simulink model "IP_order1_math_model"  (R2021a)
settings: Solver=FixedStepAuto  StartTime=0.0  StopTime=10  FixedStep=1e-4  RelTol=1e-4
values from neighbouring files (symbols this model uses):
  g = 9.8    [main_order1.m]
  I = m*l^2/3    (= 0.0166666666667)    [main_order1.m]
  K = K_lqr    [main_order1.m]
  K_lqr = lqr(A,B,Q,R)    [main_order1.m]
  l = 0.5    [main_order1.m]
  m = A_k * m +C_k    [SolveLinearMPC.m]    (also in main_order1.m = 0.2)
  M = cell2mat(M)    [SolveLinearMPC.m]    (also in main_order1.m = 0.6)
libraries: pid_lib x2
settings Model: Creator=cc  LastModifiedBy=zyinx

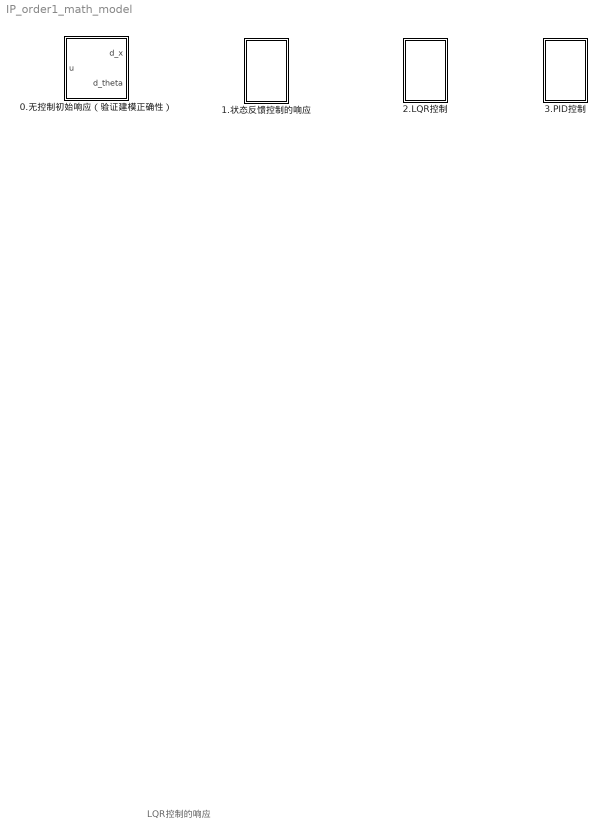
== system IP_order1_math_model ==
  note: LQR控制的响应
  0.无控制初始响应（验证建模正确性） : Subsystem
  1.状态反馈控制的响应 : Subsystem
  2.LQR控制 : Subsystem
  3.PID控制 : Subsystem

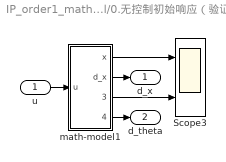
== system IP_order1_math_model/0.无控制初始响应（验证建模正确性） ==
  u : Inport
  Scope3 : Scope  NumInputPorts=2
  math-model1 : Subsystem  mask{theta_0=30/180*pi, x_0=0}
  d_x : Outport
  d_theta : Outport  Port=2
  wires:
  math-model1/2(d_x) -> d_x/1
  math-model1/1(x) -> Scope3/1
  math-model1/3(theta) -> Scope3/2
  math-model1/4(d_theta) -> d_theta/1
  u/1 -> math-model1/1(u)

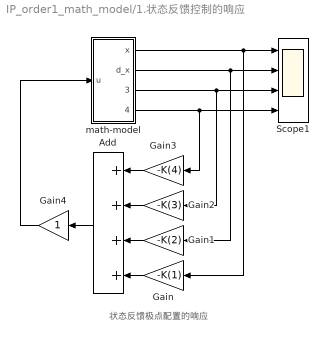
== system IP_order1_math_model/1.状态反馈控制的响应 ==
  note: 状态反馈极点配置的响应
  Add : Sum  Inputs=++++
  Gain : Gain  Gain=-K(1)
  Gain1 : Gain  Gain=-K(2)
  Gain2 : Gain  Gain=-K(3)
  Gain3 : Gain  Gain=-K(4)
  Gain4 : Gain
  Scope1 : Scope  NumInputPorts=4
  math-model : Subsystem  mask{theta_0=5/180*pi, x_0=0}
  wires:
  math-model/2(d_x) -> Gain1/1, Scope1/2
  math-model/3(theta) -> Scope1/3, Gain2/1
  math-model/1(x) -> Gain/1, Scope1/1
  Gain3/1 -> Add/1
  Gain2/1 -> Add/2
  Gain4/1 -> math-model/1(u)
  math-model/4(d_theta) -> Scope1/4, Gain3/1
  Gain/1 -> Add/4
  Gain1/1 -> Add/3
  Add/1 -> Gain4/1

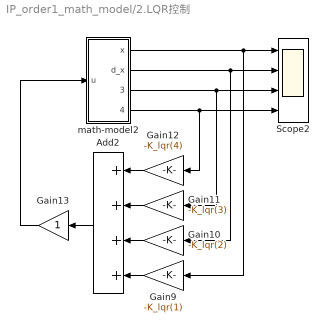
== system IP_order1_math_model/2.LQR控制 ==
  Add2 : Sum  Inputs=++++
  Gain10 : Gain  Gain=-K_lqr(2)
  Gain11 : Gain  Gain=-K_lqr(3)
  Gain12 : Gain  Gain=-K_lqr(4)
  Gain13 : Gain
  Gain9 : Gain  Gain=-K_lqr(1)
  Scope2 : Scope  NumInputPorts=4
  math-model2 : Subsystem  mask{theta_0=5/180*pi, x_0=0}
  wires:
  Gain13/1 -> math-model2/1(u)
  math-model2/2(d_x) -> Gain10/1, Scope2/2
  Gain9/1 -> Add2/4
  math-model2/3(theta) -> Scope2/3, Gain11/1
  math-model2/4(d_theta) -> Scope2/4, Gain12/1
  Add2/1 -> Gain13/1
  Gain11/1 -> Add2/2
  Gain12/1 -> Add2/1
  math-model2/1(x) -> Gain9/1, Scope2/1
  Gain10/1 -> Add2/3

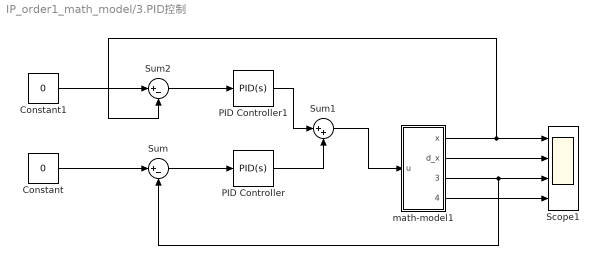
== system IP_order1_math_model/3.PID控制 ==
  Constant : Constant  Value=0
  Constant1 : Constant  Value=0
  PID Controller : pid_lib/PID Controller  Controller=PID  Form=Parallel  TimeDomain=Continuous-time  UseExternalTs=off  SampleTime=-1  IntegratorMethod=Forward Euler  FilterMethod=Forward Euler  ControllerParametersSource=internal  P=-71.4862227329796  I=-56.1535498501713  D=-22.3465648631761  UseFilter=on  N=91.5133935447898  TunerSelectOption=Transfer Function Based (PID Tuner App)  InitialConditionSource=internal  InitialConditionForIntegrator=0  InitialConditionForFilter=0  DifferentiatorICPrevScaledInput=0  ExternalReset=none  TrackingMode=off  Kt=1  LimitOutput=off  SatLimitsSource=internal  UpperSaturationLimit=inf  LowerSaturationLimit=-inf  LinearizeAsGain=on  AntiWindupMode=none  Kb=1  POutMin=[]  POutMax=[]  IOutMin=[]  IOutMax=[]  DOutMin=[]  DOutMax=[]  NOutMin=[]  NOutMax=[]  SumOutMin=[]  SumOutMax=[]  SaturationOutMin=[]  SaturationOutMax=[]  PParamMin=[]  PParamMax=[]  IParamMin=[]  IParamMax=[]  DParamMin=[]  DParamMax=[]  NParamMin=[]  NParamMax=[]  KbParamMin=[]  KbParamMax=[]  KtParamMin=[]  KtParamMax=[]  KbOutMin=[]  KbOutMax=[]  KtOutMin=[]  KtOutMax=[]  IntegratorOutMin=[]  IntegratorOutMax=[]  FilterOutMin=[]  FilterOutMax=[]  SumI1OutMin=[]  SumI1OutMax=[]  SumI2OutMin=[]  SumI2OutMax=[]  SumI3OutMin=[]  SumI3OutMax=[]  SumI4OutMin=[]  SumI4OutMax=[]  SumDOutMin=[]  SumDOutMax=[]  DifferentiatorOutMin=[]  DifferentiatorOutMax=[]  FilterDiffOutCoefMin=[]  FilterDiffOutCoefMax=[]  ReciprocalOutMin=[]  ReciprocalOutMax=[]  SumDenOutMin=[]  SumDenOutMax=[]  SumNumOutMin=[]  SumNumOutMax=[]  DivideOutMin=[]  DivideOutMax=[]  UdiffTsProdOutMin=[]  UdiffTsProdOutMax=[]  NTsProdOutMin=[]  NTsProdOutMax=[]  UintegralTsProdOutMin=[]  UintegralTsProdOutMax=[]  UngainTsProdOutMin=[]  UngainTsProdOutMax=[]  IntegratorContinuousStateAttributes=''  IntegratorStateMustResolveToSignalObject=off  IntegratorRTWStateStorageClass=Auto  FilterContinuousStateAttributes=''  FilterStateMustResolveToSignalObject=off  FilterRTWStateStorageClass=Auto  ParallelPVariant=InternalParameters  IdealPVariant=Disabled  IVariant=InternalParameters  DVariant=InternalParameters  IntegratorVariant=Continuous  SatVariant=Disabled  AWVariant=Passthrough  PCopyVariant=Disabled  TRVariant=Disabled  FdbkBlocksVariant=Forward  IdealPFdbkVariant=Disabled  SatFdbkVariant=Disabled  DerivativeFilterVariant=ContFilter  NVariant=InternalParameters  NCopyVariant=Disabled  FilterICVariant=InternalICsFilter  IntegratorICVariant=InternalICs  ExternalResetVariant=Disabled  TRSumVariant=Passthrough  SumFdbkVariant=Disabled  SumVariant=Sum_PID  TsampFilterVariant=InternalTs  TsampNgainVariant=Passthrough  TsampIntegralVariant=Passthrough  ExternalSaturationOutDataTypeStr=Inherit: Same as second input
  PID Controller1 : pid_lib/PID Controller  Controller=PID  Form=Parallel  TimeDomain=Continuous-time  UseExternalTs=off  SampleTime=-1  IntegratorMethod=Forward Euler  FilterMethod=Forward Euler  ControllerParametersSource=internal  P=-0.651476139628385  I=-0.0254147413614223  D=0.0268358303366138  UseFilter=on  N=24.2763548381633  TunerSelectOption=Transfer Function Based (PID Tuner App)  InitialConditionSource=internal  InitialConditionForIntegrator=0  InitialConditionForFilter=0  DifferentiatorICPrevScaledInput=0  ExternalReset=none  TrackingMode=off  Kt=1  LimitOutput=off  SatLimitsSource=internal  UpperSaturationLimit=inf  LowerSaturationLimit=-inf  LinearizeAsGain=on  AntiWindupMode=none  Kb=1  POutMin=[]  POutMax=[]  IOutMin=[]  IOutMax=[]  DOutMin=[]  DOutMax=[]  NOutMin=[]  NOutMax=[]  SumOutMin=[]  SumOutMax=[]  SaturationOutMin=[]  SaturationOutMax=[]  PParamMin=[]  PParamMax=[]  IParamMin=[]  IParamMax=[]  DParamMin=[]  DParamMax=[]  NParamMin=[]  NParamMax=[]  KbParamMin=[]  KbParamMax=[]  KtParamMin=[]  KtParamMax=[]  KbOutMin=[]  KbOutMax=[]  KtOutMin=[]  KtOutMax=[]  IntegratorOutMin=[]  IntegratorOutMax=[]  FilterOutMin=[]  FilterOutMax=[]  SumI1OutMin=[]  SumI1OutMax=[]  SumI2OutMin=[]  SumI2OutMax=[]  SumI3OutMin=[]  SumI3OutMax=[]  SumI4OutMin=[]  SumI4OutMax=[]  SumDOutMin=[]  SumDOutMax=[]  DifferentiatorOutMin=[]  DifferentiatorOutMax=[]  FilterDiffOutCoefMin=[]  FilterDiffOutCoefMax=[]  ReciprocalOutMin=[]  ReciprocalOutMax=[]  SumDenOutMin=[]  SumDenOutMax=[]  SumNumOutMin=[]  SumNumOutMax=[]  DivideOutMin=[]  DivideOutMax=[]  UdiffTsProdOutMin=[]  UdiffTsProdOutMax=[]  NTsProdOutMin=[]  NTsProdOutMax=[]  UintegralTsProdOutMin=[]  UintegralTsProdOutMax=[]  UngainTsProdOutMin=[]  UngainTsProdOutMax=[]  IntegratorContinuousStateAttributes=''  IntegratorStateMustResolveToSignalObject=off  IntegratorRTWStateStorageClass=Auto  FilterContinuousStateAttributes=''  FilterStateMustResolveToSignalObject=off  FilterRTWStateStorageClass=Auto  ParallelPVariant=InternalParameters  IdealPVariant=Disabled  IVariant=InternalParameters  DVariant=InternalParameters  IntegratorVariant=Continuous  SatVariant=Disabled  AWVariant=Passthrough  PCopyVariant=Disabled  TRVariant=Disabled  FdbkBlocksVariant=Forward  IdealPFdbkVariant=Disabled  SatFdbkVariant=Disabled  DerivativeFilterVariant=ContFilter  NVariant=InternalParameters  NCopyVariant=Disabled  FilterICVariant=InternalICsFilter  IntegratorICVariant=InternalICs  ExternalResetVariant=Disabled  TRSumVariant=Passthrough  SumFdbkVariant=Disabled  SumVariant=Sum_PID  TsampFilterVariant=InternalTs  TsampNgainVariant=Passthrough  TsampIntegralVariant=Passthrough  ExternalSaturationOutDataTypeStr=Inherit: Same as second input
  Scope1 : Scope  NumInputPorts=4
  Sum : Sum  Inputs=|+-
  Sum1 : Sum  Inputs=|++
  Sum2 : Sum  Inputs=|+-
  math-model1 : Subsystem  mask{theta_0=5/180*pi, x_0=0}
  wires:
  PID Controller/1 -> Sum1/2
  math-model1/2(d_x) -> Scope1/2
  math-model1/3(theta) -> Sum/2, Scope1/3
  math-model1/4(d_theta) -> Scope1/4
  Constant/1 -> Sum/1
  Sum/1 -> PID Controller/1
  PID Controller1/1 -> Sum1/1
  Sum1/1 -> math-model1/1(u)
  math-model1/1(x) -> Scope1/1, Sum2/2
  Sum2/1 -> PID Controller1/1
  Constant1/1 -> Sum2/1

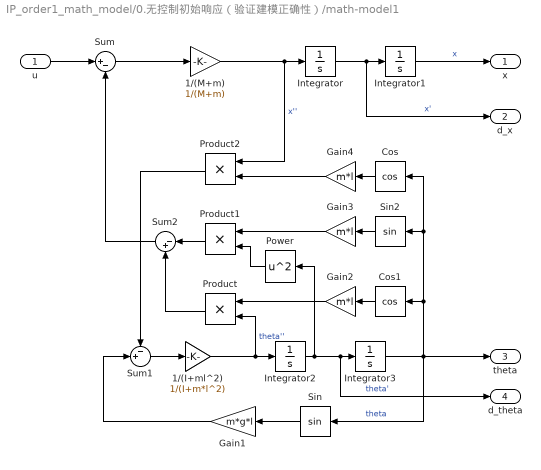
== system IP_order1_math_model/0.无控制初始响应（验证建模正确性）/math-model1 ==
  u : Inport
  1/(I+ml^2) : Gain  Gain=1/(I+m*l^2)
  1/(M+m) : Gain  Gain=1/(M+m)
  Cos : Trigonometry  Operator=cos
  Cos1 : Trigonometry  Operator=cos
  Gain1 : Gain  Gain=m*g*l
  Gain2 : Gain  Gain=m*l
  Gain3 : Gain  Gain=m*l
  Gain4 : Gain  Gain=m*l
  Integrator : Integrator
  Integrator1 : Integrator  InitialCondition=x_0
  Integrator2 : Integrator
  Integrator3 : Integrator  InitialCondition=theta_0
  Power : Math  Operator=square  SaturateOnIntegerOverflow=on
  Product : Product
  Product1 : Product
  Product2 : Product
  Sin : Trigonometry
  Sin2 : Trigonometry
  Sum : Sum  Inputs=|+-
  Sum1 : Sum  Inputs=-+|
  Sum2 : Sum  Inputs=|-+
  x : Outport  VectorParamsAs1DForOutWhenUnconnected=off
  d_x : Outport  Port=2  VectorParamsAs1DForOutWhenUnconnected=off
  theta : Outport  Port=3  VectorParamsAs1DForOutWhenUnconnected=off
  d_theta : Outport  Port=4  VectorParamsAs1DForOutWhenUnconnected=off
  wires:
  Sum/1 -> 1/(M+m)/1
  Product2/1 -> Sum1/1
  Cos1/1 -> Gain2/1
  Product1/1 -> Sum2/1
  1/(M+m)/1 -> Product2/1, Integrator/1  "x''"
  Sin/1 -> Gain1/1
  u/1 -> Sum/1
  Gain2/1 -> Product/1
  1/(I+ml^2)/1 -> Product/2, Integrator2/1  "theta''"
  Integrator3/1 -> theta/1, Cos/1, Sin2/1, Cos1/1, Sin/1  "theta"
  Integrator2/1 -> d_theta/1, Integrator3/1, Power/1  "theta'"
  Gain1/1 -> Sum1/2
  Integrator/1 -> d_x/1, Integrator1/1  "x'"
  Gain4/1 -> Product2/2
  Gain3/1 -> Product1/1
  Power/1 -> Product1/2
  Sum1/1 -> 1/(I+ml^2)/1
  Integrator1/1 -> x/1  "x"
  Sum2/1 -> Sum/2
  Product/1 -> Sum2/2
  Cos/1 -> Gain4/1
  Sin2/1 -> Gain3/1

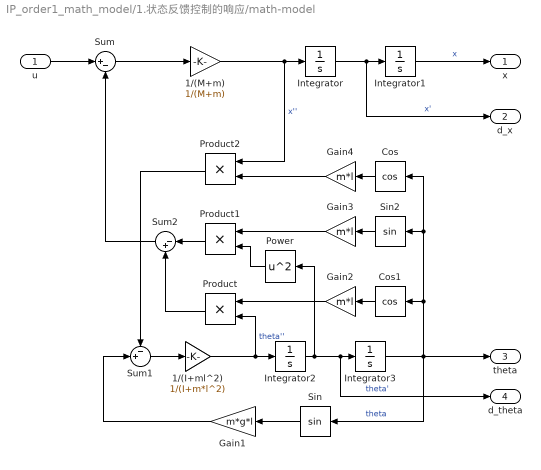
== system IP_order1_math_model/1.状态反馈控制的响应/math-model ==
  u : Inport
  1/(I+ml^2) : Gain  Gain=1/(I+m*l^2)
  1/(M+m) : Gain  Gain=1/(M+m)
  Cos : Trigonometry  Operator=cos
  Cos1 : Trigonometry  Operator=cos
  Gain1 : Gain  Gain=m*g*l
  Gain2 : Gain  Gain=m*l
  Gain3 : Gain  Gain=m*l
  Gain4 : Gain  Gain=m*l
  Integrator : Integrator
  Integrator1 : Integrator  InitialCondition=x_0
  Integrator2 : Integrator
  Integrator3 : Integrator  InitialCondition=theta_0
  Power : Math  Operator=square  SaturateOnIntegerOverflow=on
  Product : Product
  Product1 : Product
  Product2 : Product
  Sin : Trigonometry
  Sin2 : Trigonometry
  Sum : Sum  Inputs=|+-
  Sum1 : Sum  Inputs=-+|
  Sum2 : Sum  Inputs=|-+
  x : Outport  VectorParamsAs1DForOutWhenUnconnected=off
  d_x : Outport  Port=2  VectorParamsAs1DForOutWhenUnconnected=off
  theta : Outport  Port=3  VectorParamsAs1DForOutWhenUnconnected=off
  d_theta : Outport  Port=4  VectorParamsAs1DForOutWhenUnconnected=off
  wires:
  Sum/1 -> 1/(M+m)/1
  Product2/1 -> Sum1/1
  Cos1/1 -> Gain2/1
  Product1/1 -> Sum2/1
  1/(M+m)/1 -> Product2/1, Integrator/1  "x''"
  Sin/1 -> Gain1/1
  u/1 -> Sum/1
  Gain2/1 -> Product/1
  1/(I+ml^2)/1 -> Product/2, Integrator2/1  "theta''"
  Integrator3/1 -> theta/1, Cos/1, Sin2/1, Cos1/1, Sin/1  "theta"
  Integrator2/1 -> d_theta/1, Integrator3/1, Power/1  "theta'"
  Gain1/1 -> Sum1/2
  Integrator/1 -> d_x/1, Integrator1/1  "x'"
  Gain4/1 -> Product2/2
  Gain3/1 -> Product1/1
  Power/1 -> Product1/2
  Sum1/1 -> 1/(I+ml^2)/1
  Integrator1/1 -> x/1  "x"
  Sum2/1 -> Sum/2
  Product/1 -> Sum2/2
  Cos/1 -> Gain4/1
  Sin2/1 -> Gain3/1

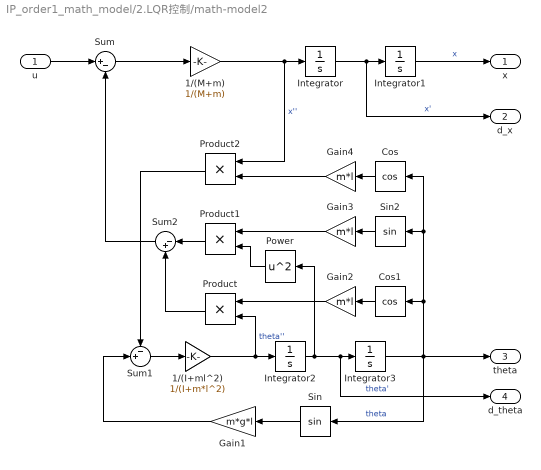
== system IP_order1_math_model/2.LQR控制/math-model2 ==
  u : Inport
  1/(I+ml^2) : Gain  Gain=1/(I+m*l^2)
  1/(M+m) : Gain  Gain=1/(M+m)
  Cos : Trigonometry  Operator=cos
  Cos1 : Trigonometry  Operator=cos
  Gain1 : Gain  Gain=m*g*l
  Gain2 : Gain  Gain=m*l
  Gain3 : Gain  Gain=m*l
  Gain4 : Gain  Gain=m*l
  Integrator : Integrator
  Integrator1 : Integrator  InitialCondition=x_0
  Integrator2 : Integrator
  Integrator3 : Integrator  InitialCondition=theta_0
  Power : Math  Operator=square  SaturateOnIntegerOverflow=on
  Product : Product
  Product1 : Product
  Product2 : Product
  Sin : Trigonometry
  Sin2 : Trigonometry
  Sum : Sum  Inputs=|+-
  Sum1 : Sum  Inputs=-+|
  Sum2 : Sum  Inputs=|-+
  x : Outport  VectorParamsAs1DForOutWhenUnconnected=off
  d_x : Outport  Port=2  VectorParamsAs1DForOutWhenUnconnected=off
  theta : Outport  Port=3  VectorParamsAs1DForOutWhenUnconnected=off
  d_theta : Outport  Port=4  VectorParamsAs1DForOutWhenUnconnected=off
  wires:
  Sum/1 -> 1/(M+m)/1
  Product2/1 -> Sum1/1
  Cos1/1 -> Gain2/1
  Product1/1 -> Sum2/1
  1/(M+m)/1 -> Product2/1, Integrator/1  "x''"
  Sin/1 -> Gain1/1
  u/1 -> Sum/1
  Gain2/1 -> Product/1
  1/(I+ml^2)/1 -> Product/2, Integrator2/1  "theta''"
  Integrator3/1 -> theta/1, Cos/1, Sin2/1, Cos1/1, Sin/1  "theta"
  Integrator2/1 -> d_theta/1, Integrator3/1, Power/1  "theta'"
  Gain1/1 -> Sum1/2
  Integrator/1 -> d_x/1, Integrator1/1  "x'"
  Gain4/1 -> Product2/2
  Gain3/1 -> Product1/1
  Power/1 -> Product1/2
  Sum1/1 -> 1/(I+ml^2)/1
  Integrator1/1 -> x/1  "x"
  Sum2/1 -> Sum/2
  Product/1 -> Sum2/2
  Cos/1 -> Gain4/1
  Sin2/1 -> Gain3/1

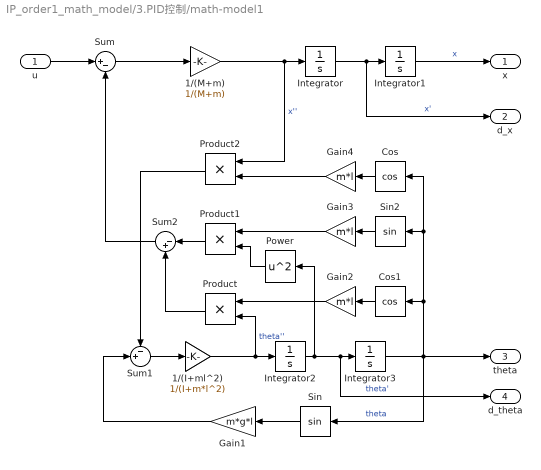
== system IP_order1_math_model/3.PID控制/math-model1 ==
  u : Inport
  1/(I+ml^2) : Gain  Gain=1/(I+m*l^2)
  1/(M+m) : Gain  Gain=1/(M+m)
  Cos : Trigonometry  Operator=cos
  Cos1 : Trigonometry  Operator=cos
  Gain1 : Gain  Gain=m*g*l
  Gain2 : Gain  Gain=m*l
  Gain3 : Gain  Gain=m*l
  Gain4 : Gain  Gain=m*l
  Integrator : Integrator
  Integrator1 : Integrator  InitialCondition=x_0
  Integrator2 : Integrator
  Integrator3 : Integrator  InitialCondition=theta_0
  Power : Math  Operator=square  SaturateOnIntegerOverflow=on
  Product : Product
  Product1 : Product
  Product2 : Product
  Sin : Trigonometry
  Sin2 : Trigonometry
  Sum : Sum  Inputs=|+-
  Sum1 : Sum  Inputs=-+|
  Sum2 : Sum  Inputs=|-+
  x : Outport  VectorParamsAs1DForOutWhenUnconnected=off
  d_x : Outport  Port=2  VectorParamsAs1DForOutWhenUnconnected=off
  theta : Outport  Port=3  VectorParamsAs1DForOutWhenUnconnected=off
  d_theta : Outport  Port=4  VectorParamsAs1DForOutWhenUnconnected=off
  wires:
  Sum/1 -> 1/(M+m)/1
  Product2/1 -> Sum1/1
  Cos1/1 -> Gain2/1
  Product1/1 -> Sum2/1
  1/(M+m)/1 -> Product2/1, Integrator/1  "x''"
  Sin/1 -> Gain1/1
  u/1 -> Sum/1
  Gain2/1 -> Product/1
  1/(I+ml^2)/1 -> Product/2, Integrator2/1  "theta''"
  Integrator3/1 -> theta/1, Cos/1, Sin2/1, Cos1/1, Sin/1  "theta"
  Integrator2/1 -> d_theta/1, Integrator3/1, Power/1  "theta'"
  Gain1/1 -> Sum1/2
  Integrator/1 -> d_x/1, Integrator1/1  "x'"
  Gain4/1 -> Product2/2
  Gain3/1 -> Product1/1
  Power/1 -> Product1/2
  Sum1/1 -> 1/(I+ml^2)/1
  Integrator1/1 -> x/1  "x"
  Sum2/1 -> Sum/2
  Product/1 -> Sum2/2
  Cos/1 -> Gain4/1
  Sin2/1 -> Gain3/1
